simulink model "Quadrotor"  (R2020b)
settings: Solver=FixedStepAuto  StartTime=0.0  StopTime=10.0  FixedStep=1e-4  RelTol=1e-3
settings Model: Creator=贺嘉辣  LastModifiedBy=贺嘉辣

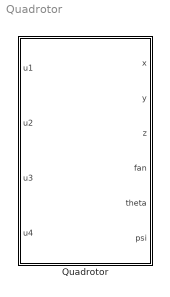
== system Quadrotor ==
  Quadrotor : Subsystem  mask{m=0.65, g=9.8, Ixx=7.5e-3, Iyy=7.5e-3, Izz=1.3e-2, L=0.23, rho=3.1e-5, gama=7.5e-7}
      mask prompts: m "无人机质量"; g "重力加速度"; Ixx "四旋翼绕X轴转动惯量"; Iyy "四旋翼绕Y轴转动惯量"; Izz "四旋翼绕Z轴转动惯量"; L "四旋翼臂长"; rho "四旋翼升力系数"; gama "空气阻力系数"

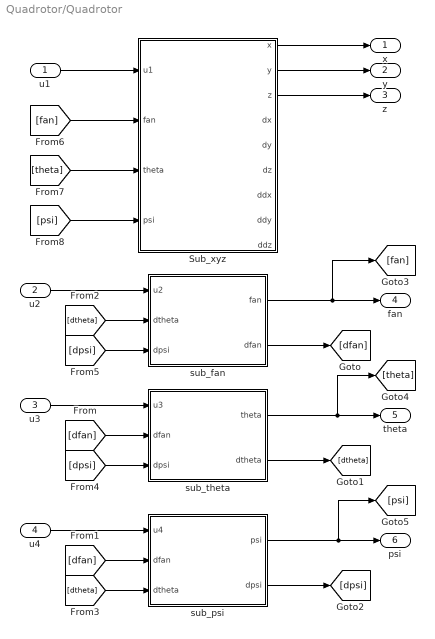
== system Quadrotor/Quadrotor ==
  u1 : Inport
  u2 : Inport  Port=2
  u3 : Inport  Port=3
  u4 : Inport  Port=4
  Sub_xyz : Subsystem
  sub_fan : Subsystem
  sub_psi : Subsystem
  sub_theta : Subsystem
  x : Outport
  y : Outport  Port=2
  z : Outport  Port=3
  fan : Outport  Port=4
  theta : Outport  Port=5
  psi : Outport  Port=6
  wires:
  u2/1 -> sub_fan/1(u2)
  u3/1 -> sub_theta/1(u3)
  u4/1 -> sub_psi/1(u4)
  sub_fan/1(fan) -> [fan], fan/1
  sub_theta/1(theta) -> [theta], theta/1
  sub_psi/1(psi) -> [psi], psi/1
  sub_fan/2(dfan) -> [dfan]
  [dfan] -> sub_theta/2(dfan)
  [dfan] -> sub_psi/2(dfan)
  sub_theta/2(dtheta) -> [dtheta]
  sub_psi/2(dpsi) -> [dpsi]
  [dtheta] -> sub_fan/2(dtheta)
  [dtheta] -> sub_psi/3(dtheta)
  [dpsi] -> sub_theta/3(dpsi)
  [dpsi] -> sub_fan/3(dpsi)
  u1/1 -> Sub_xyz/1(u1)
  Sub_xyz/1(x) -> x/1
  Sub_xyz/2(y) -> y/1
  Sub_xyz/3(z) -> z/1
  [fan] -> Sub_xyz/2(fan)
  [theta] -> Sub_xyz/3(theta)
  [psi] -> Sub_xyz/4(psi)

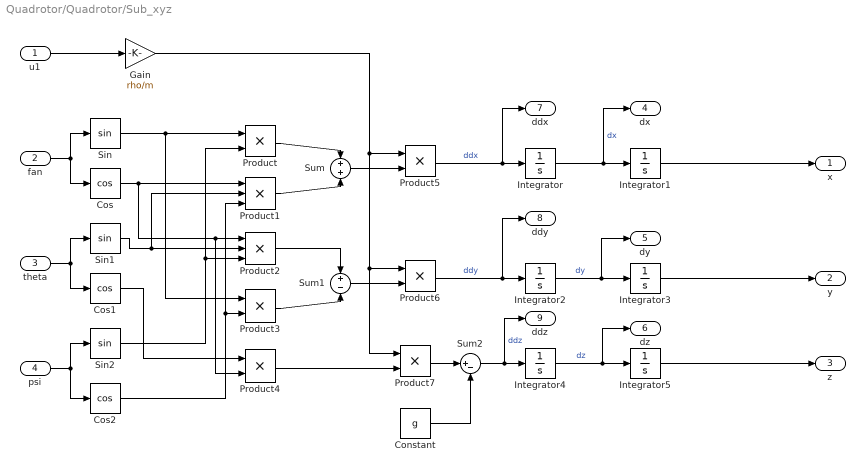
== system Quadrotor/Quadrotor/Sub_xyz ==
  u1 : Inport
  fan : Inport  Port=2
  theta : Inport  Port=3
  psi : Inport  Port=4
  Constant : Constant  Value=g
  Cos : Trigonometry  Operator=cos
  Cos1 : Trigonometry  Operator=cos
  Cos2 : Trigonometry  Operator=cos
  Gain : Gain  Gain=rho/m
  Integrator{,1..5} (6 alike) : Integrator
  Product{,3..7} (6 alike) : Product
  Product1 : Product  Inputs=3
  Product2 : Product  Inputs=3
  Sin : Trigonometry
  Sin1 : Trigonometry
  Sin2 : Trigonometry
  Sum : Sum  Inputs=+|+
  Sum1 : Sum  Inputs=+|-
  Sum2 : Sum  Inputs=|+-
  x : Outport
  y : Outport  Port=2
  z : Outport  Port=3
  dx : Outport  Port=4
  dy : Outport  Port=5
  dz : Outport  Port=6
  ddx : Outport  Port=7
  ddy : Outport  Port=8
  ddz : Outport  Port=9
  wires:
  u1/1 -> Gain/1
  fan/1 -> Cos/1, Sin/1
  theta/1 -> Cos1/1, Sin1/1
  psi/1 -> Cos2/1, Sin2/1
  Sin/1 -> Product3/1, Product/1
  Sin2/1 -> Product/2, Product2/3
  Cos/1 -> Product4/2, Product2/1, Product1/1
  Sin1/1 -> Product2/2, Product1/2
  Cos2/1 -> Product1/3, Product3/2
  Product/1 -> Sum/1
  Product1/1 -> Sum/2
  Cos1/1 -> Product4/1
  Product2/1 -> Sum1/1
  Product3/1 -> Sum1/2
  Sum/1 -> Product5/2
  Sum1/1 -> Product6/2
  Product4/1 -> Product7/2
  Gain/1 -> Product7/1, Product6/1, Product5/1
  Product5/1 -> ddx/1, Integrator/1  "ddx"
  Integrator/1 -> dx/1, Integrator1/1  "dx"
  Product6/1 -> ddy/1, Integrator2/1  "ddy"
  Integrator2/1 -> dy/1, Integrator3/1  "dy"
  Product7/1 -> Sum2/1
  Constant/1 -> Sum2/2
  Sum2/1 -> ddz/1, Integrator4/1  "ddz"
  Integrator4/1 -> dz/1, Integrator5/1  "dz"
  Integrator3/1 -> y/1
  Integrator1/1 -> x/1
  Integrator5/1 -> z/1

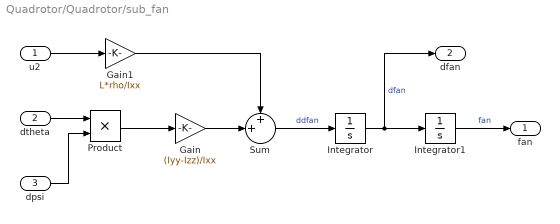
== system Quadrotor/Quadrotor/sub_fan ==
  u2 : Inport
  dtheta : Inport  Port=2
  dpsi : Inport  Port=3
  Gain : Gain  Gain=(Iyy-Izz)/Ixx
  Gain1 : Gain  Gain=L*rho/Ixx
  Integrator : Integrator
  Integrator1 : Integrator
  Product : Product
  Sum : Sum  Inputs=++|
  fan : Outport
  dfan : Outport  Port=2
  wires:
  Sum/1 -> Integrator/1  "ddfan"
  Integrator/1 -> dfan/1, Integrator1/1  "dfan"
  Integrator1/1 -> fan/1  "fan"
  dtheta/1 -> Product/1
  dpsi/1 -> Product/2
  Product/1 -> Gain/1
  Gain/1 -> Sum/2
  u2/1 -> Gain1/1
  Gain1/1 -> Sum/1

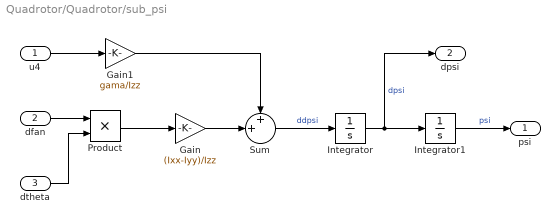
== system Quadrotor/Quadrotor/sub_psi ==
  u4 : Inport
  dfan : Inport  Port=2
  dtheta : Inport  Port=3
  Gain : Gain  Gain=(Ixx-Iyy)/Izz
  Gain1 : Gain  Gain=gama/Izz
  Integrator : Integrator
  Integrator1 : Integrator
  Product : Product
  Sum : Sum  Inputs=++|
  psi : Outport
  dpsi : Outport  Port=2
  wires:
  Sum/1 -> Integrator/1  "ddpsi"
  Integrator/1 -> dpsi/1, Integrator1/1  "dpsi"
  Integrator1/1 -> psi/1  "psi"
  dfan/1 -> Product/1
  dtheta/1 -> Product/2
  Product/1 -> Gain/1
  Gain/1 -> Sum/2
  u4/1 -> Gain1/1
  Gain1/1 -> Sum/1

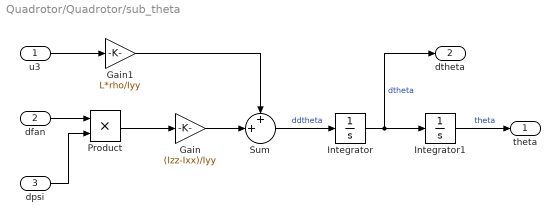
== system Quadrotor/Quadrotor/sub_theta ==
  u3 : Inport
  dfan : Inport  Port=2
  dpsi : Inport  Port=3
  Gain : Gain  Gain=(Izz-Ixx)/Iyy
  Gain1 : Gain  Gain=L*rho/Iyy
  Integrator : Integrator
  Integrator1 : Integrator
  Product : Product
  Sum : Sum  Inputs=++|
  theta : Outport
  dtheta : Outport  Port=2
  wires:
  Sum/1 -> Integrator/1  "ddtheta"
  Integrator/1 -> dtheta/1, Integrator1/1  "dtheta"
  Integrator1/1 -> theta/1  "theta"
  dfan/1 -> Product/1
  dpsi/1 -> Product/2
  Product/1 -> Gain/1
  Gain/1 -> Sum/2
  u3/1 -> Gain1/1
  Gain1/1 -> Sum/1
